simulink model "a3_margens_estabilidade_smlk"  (R2023b)
settings: Solver=VariableStepAuto  StartTime=0.0  StopTime=12  FixedStep=.02  RelTol=1e-3
values from neighbouring files (symbols this model uses):
  Kmax = 10^(20.8/20)    (= 10.9647819614)    [a3_margens_estabilidade.m]    (also in a4_.m; a4_exercicio.m)
settings Model: Creator=LUCAS  LastModifiedBy=LUCAS

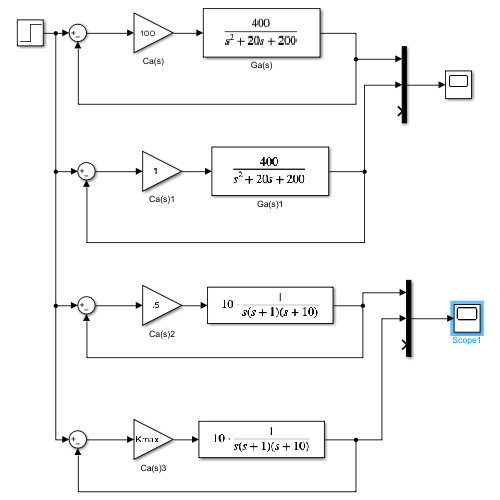
[thumbnail: Simulink's stored preview of the top-level diagram]
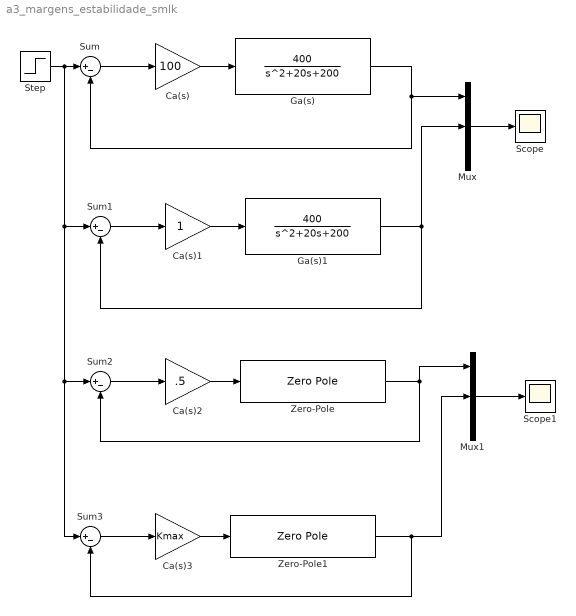
== system a3_margens_estabilidade_smlk ==
  Ca(s) : Gain  Gain=100
  Ca(s)1 : Gain
  Ca(s)2 : Gain  Gain=.5
  Ca(s)3 : Gain  Gain=Kmax
  Ga(s) : TransferFcn  Numerator=[400]  Denominator=[1 20 200]
  Ga(s)1 : TransferFcn  Numerator=[400]  Denominator=[1 20 200]
  Mux : Mux  Inputs=3
  Mux1 : Mux  Inputs=3
  Scope : Scope
  Scope1 : Scope
  Step : Step  SampleTime=0
  Sum{,1..3} (4 alike) : Sum  Inputs=|+-
  Zero-Pole : ZeroPole  Zeros=[]  Poles=[0 -1 -10]  Gain=10
  Zero-Pole1 : ZeroPole  Zeros=[]  Poles=[0 -1 -10]  Gain=10
  wires:
  Ca(s)/1 -> Ga(s)/1
  Ga(s)/1 -> Mux/1, Sum/2
  Sum/1 -> Ca(s)/1
  Step/1 -> Sum2/1, Sum3/1, Sum1/1, Sum/1
  Sum1/1 -> Ca(s)1/1
  Ca(s)1/1 -> Ga(s)1/1
  Ga(s)1/1 -> Mux/2, Sum1/2
  Mux/1 -> Scope/1
  Sum2/1 -> Ca(s)2/1
  Ca(s)2/1 -> Zero-Pole/1
  Zero-Pole/1 -> Mux1/1, Sum2/2
  Zero-Pole1/1 -> Mux1/2, Sum3/2
  Ca(s)3/1 -> Zero-Pole1/1
  Sum3/1 -> Ca(s)3/1
  Mux1/1 -> Scope1/1
